simulink model "quad_ASMC"  (R2023a)
settings: Solver=ode4  StartTime=0.0  StopTime=tf  FixedStep=0.01  RelTol=1e-3
model workspace (MAT data in the model file):
  tf = Simulink.Parameter
  tf.Value = 60
  tf.DataType = 'auto'
  tf.Complexity = 'real'
  tf.Dimensions = [1 1]
  tray2 = [0  2  2  -2  -2  0; 0  0  -2  -2  2  0; 0  5  2.5  5  2.5  0; 0  0  0  0  0  0; 0  0  0  0  0  0; 0  0  0  0  0  0]
libraries: robotcorelib x1
settings Model: Creator=adan  LastModifiedBy=Adan Daniel
settings OptimizationCC: ReuseModelBlockBuffer=off

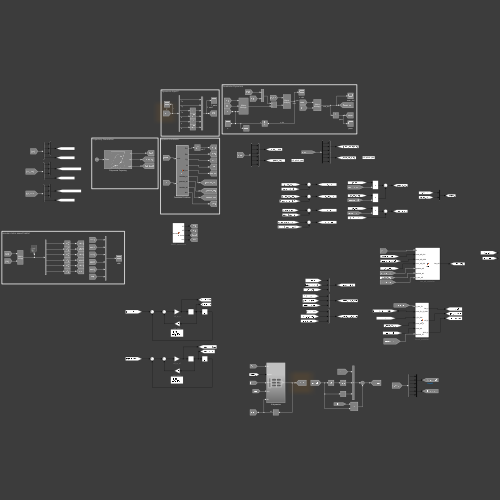
[thumbnail: Simulink's stored preview of the top-level diagram]
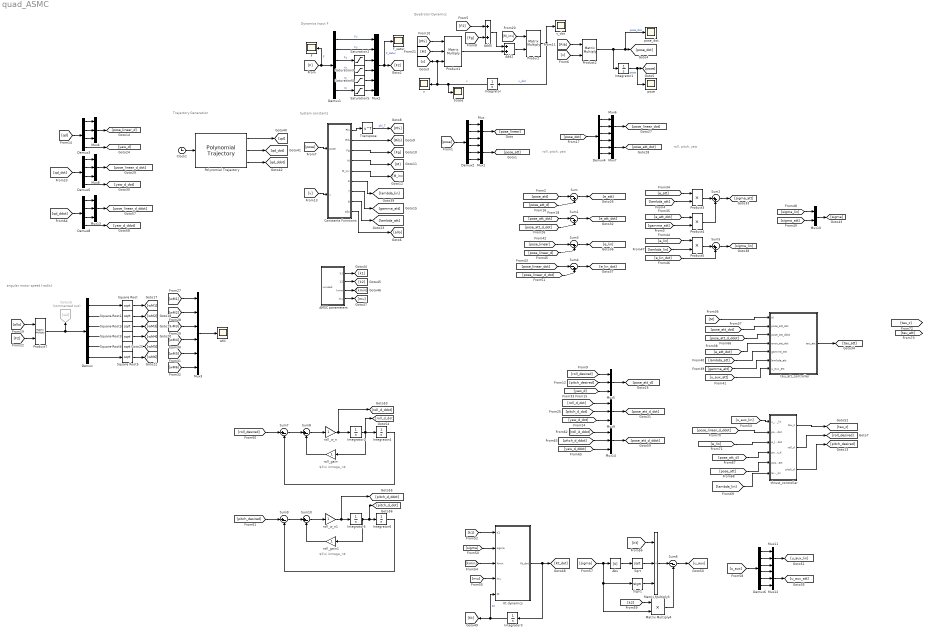
== system quad_ASMC ==
  note: $2\xi \omega_n$
  note: roll, pitch, yaw
  note: angular motor speed [rad/s]
  note: System constants
  note: Quadrotor Dynamics
  note: Dynamics Input F
  note: Trajectory Generation
  note: roll, pitch, yaw
  note: $2\xi \omega_n$
  AMSC parameters : MATLAB Function  TreatAsAtomicUnit=on
  Abs : Abs  SaturateOnIntegerOverflow=off
  Add2 : Sum
  Add5 : Sum
  Clock1 : Clock
  Constants Functions : MATLAB Function  TreatAsAtomicUnit=on
  Demux{,1..2,4,6} (5 alike) : Demux  Outputs=6
  Demux3 : Demux
  Demux5 : Demux
  Demux8 : Demux
  F : Scope
  F_satur : Scope
  Goto16 : Goto  Commented=on  GotoTag=w2
  Integrator : Integrator  InitialCondition=[0; 0; 0; 0; 0; 0]
  Integrator1 : Integrator  InitialCondition=[0; 0; 0; 0; 0; 0]
  Integrator{2,4..6} (4 alike) : Integrator
  Integrator3 : Integrator  InitialCondition=[0; 0; 0; 0; 0; 0]
  Kt dynamics : Subsystem
  Matrix Multiply3 : Product  Inputs=3
  Matrix Multiply4 : Product
  Mux{,1,4..9,11..14} (12 alike) : Mux  Inputs=3
  Mux10 : Mux  Inputs=2
  Mux2 : Mux  Inputs=6
  Mux3 : Mux  Inputs=6
  Polynomial Trajectory : robotcorelib/Polynomial Trajectory  WaypointSource=Internal  Waypoints=tray2  TimePoints=[ 0, 12, 24, 35, 48, tf ]  TimeInterval=[ 1, 4 ]  Method=Cubic Polynomial  ParameterSource=Internal  VelocityBoundaryCondition=zeros( 6, 6 )  AccelerationBoundaryCondition=zeros( 2, 5 )  SimulateUsing=Interpreted execution
  Product : Product  Multiplication=Matrix(*)
  Product1 : Product  Inputs=3  Multiplication=Matrix(*)
  Product2 : Product  Multiplication=Matrix(*)
  Product3 : Product
  Product4 : Product
  Product5 : Product
  Product7 : Product  Multiplication=Matrix(*)
  Saturation2 : Saturate  UpperLimit=5.8*6  LowerLimit=0
  Saturation3 : Saturate
  Saturation4 : Saturate
  Saturation5 : Saturate
  Scope : Scope
  Sign1 : Signum
  Sqrt : Sqrt
  Square Root{,1..5} (6 alike) : Sqrt
  Sum{,1,3..4} (4 alike) : Sum  Inputs=|-+
  Sum{7..10} (4 alike) : Sum  Inputs=|+-
  Sum2 : Sum  Inputs=|++
  Sum5 : Sum  Inputs=|++
  Sum6 : Sum  Inputs=|--
  Transpose : Math  Operator=transpose
  pose : Scope
  pose_dot : Scope
  roll_gain : Gain
  roll_gain1 : Gain
  roll_w_n : Gain
  roll_w_n1 : Gain
  tau_att_controller : MATLAB Function  TreatAsAtomicUnit=on
  thrust_controller : MATLAB Function  TreatAsAtomicUnit=on
  v : Scope
  v_dot : Scope
  wMi : Scope
  wires:
  Saturation4/1 -> Mux2/5
  Saturation3/1 -> Mux2/4
  Demux1/6 -> Saturation5/1  "tz"
  Demux1/3 -> Saturation2/1  "Fz"
  [F] -> F/1, Demux1/1  "F"
  Saturation5/1 -> Mux2/6
  Demux1/2 -> Mux2/2  "Fy"
  Demux1/1 -> Mux2/1  "Fx"
  Demux1/5 -> Saturation4/1  "ty"
  Demux1/4 -> Saturation3/1  "tx"
  Saturation2/1 -> Mux2/3
  Mux2/1 -> F_satur/1, [F2]  "F_satur"
  [M] -> Product1/2
  [v] -> Product2/2
  [M_inv] -> Product/1
  Add2/1 -> Product/2
  Product/1 -> v_dot/1, Integrator/1  "v_dot"
  [Rib] -> Product2/1
  Product2/1 -> Integrator1/1, pose_dot/1, [pose_dot]  "pose_dot"
  [Phi] -> Product1/1
  Product1/1 -> Add2/2
  Integrator1/1 -> pose/1, [pose]  "pose"
  Integrator/1 -> Scope/1, v/1, [v], Product1/3  "v"
  [Fg] -> Add5/2
  Add5/1 -> Add2/1
  [F2] -> Add5/1
  Constants Functions/1(Phi) -> Transpose/1
  Constants Functions/3(Fg) -> [Fg]
  Constants Functions/2(Rib) -> [Rib]
  Transpose/1 -> [Phi]  "phi_T"
  Constants Functions/5(M_inv) -> [M_inv]
  Constants Functions/4(M) -> [M]
  Constants Functions/9(allo) -> [allo]
  [v] -> Constants Functions/2(v)
  [pose] -> Constants Functions/1(pose)
  [wM3] -> Mux3/3
  [allo] -> Product7/1
  [wM6] -> Mux3/6
  [wM2] -> Mux3/2
  Demux/2 -> Square Root1/1
  Product7/1 -> Demux/1, Goto16/1
  Demux/6 -> Square Root5/1
  Demux/5 -> Square Root4/1
  [wM4] -> Mux3/4
  Mux3/1 -> wMi/1
  Square Root2/1 -> [wM3]
  Demux/4 -> Square Root3/1
  Demux/1 -> Square Root/1
  [wM1] -> Mux3/1
  [F2] -> Product7/2
  Square Root1/1 -> [wM2]
  [wM5] -> Mux3/5
  Square Root4/1 -> [wM5]
  Demux/3 -> Square Root2/1
  Square Root5/1 -> [wM6]
  Square Root3/1 -> [wM4]
  Square Root/1 -> [wM1]
  Polynomial Trajectory/1 -> [qd]
  Clock1/1 -> Polynomial Trajectory/1
  Polynomial Trajectory/2 -> [qd_dot]
  Polynomial Trajectory/3 -> [qd_ddot]
  Constants Functions/7(gamma_att) -> [gamma_att]
  Constants Functions/8(lambda_att) -> [lambda_att]
  [pose] -> Demux2/1
  Demux2/3 -> Mux/3
  Demux2/2 -> Mux/2
  Demux2/1 -> Mux/1
  Demux2/4 -> Mux1/1
  Demux2/5 -> Mux1/2
  Demux2/6 -> Mux1/3
  Mux/1 -> [pose_linear]
  Mux1/1 -> [pose_att]
  [qd] -> Demux3/1
  Demux3/3 -> Mux4/3
  Demux3/2 -> Mux4/2
  Demux3/1 -> Mux4/1
  Mux4/1 -> [pose_linear_d]
  Demux3/4 -> [yaw_d]
  [yaw_d] -> Mux5/3
  [pitch_desired] -> Mux5/2
  [roll_desired] -> Mux5/1
  Mux5/1 -> [pose_att_d]
  [pose_att] -> Sum/1
  [pose_att_d] -> Sum/2
  Sum/1 -> [e_att]
  Mux7/1 -> [pose_att_dot]
  Demux4/6 -> Mux7/3
  [pose_dot] -> Demux4/1
  Demux4/1 -> Mux6/1
  Demux4/2 -> Mux6/2
  Demux4/5 -> Mux7/2
  Demux4/4 -> Mux7/1
  Mux6/1 -> [pose_linear_dot]
  Demux4/3 -> Mux6/3
  Demux5/2 -> Mux8/2
  Mux8/1 -> [pose_linear_d_dot]
  Demux5/4 -> [yaw_d_dot]
  [qd_dot] -> Demux5/1
  Demux5/3 -> Mux8/3
  Demux5/1 -> Mux8/1
  [pitch_d_dot] -> Mux9/2
  [yaw_d_dot] -> Mux9/3
  Mux9/1 -> [pose_att_d_dot]
  [roll_d_dot] -> Mux9/1
  [pose_att_d_dot] -> Sum1/2
  [pose_att_dot] -> Sum1/1
  Sum1/1 -> [e_att_dot]
  [e_att] -> Product3/1
  [lambda_att] -> Product3/2
  [gamma_att] -> Product4/2
  [e_att_dot] -> Product4/1
  Product3/1 -> Sum2/1
  Product4/1 -> Sum2/2
  Sum2/1 -> [sigma_att]
  [M] -> tau_att_controller/1(M)
  [pose_att_dot] -> tau_att_controller/2(pose_att_dot)
  [e_att_dot] -> tau_att_controller/4(error_att_dot)
  [lambda_att] -> tau_att_controller/5(gamma_att)
  [gamma_att] -> tau_att_controller/6(lambda_att)
  [u_aux_att] -> tau_att_controller/7(u_aux_att)
  tau_att_controller/1(tau_att) -> [tau_att]
  Sum4/1 -> [e_lin_dot]
  [e_lin_dot] -> Sum5/2
  [pose_linear_d] -> Sum3/2
  [lambda_lin] -> Product5/2
  [e_lin] -> Product5/1
  [pose_linear_dot] -> Sum4/1
  [pose_linear_d_dot] -> Sum4/2
  Product5/1 -> Sum5/1
  [pose_linear] -> Sum3/1
  Sum5/1 -> [sigma_lin]
  Sum3/1 -> [e_lin]
  Constants Functions/6(lambda_lin) -> [lambda_lin]
  [sigma_lin] -> Mux10/1
  [sigma_att] -> Mux10/2
  Mux10/1 -> [sigma]
  AMSC parameters/1(k1) -> [k1]
  AMSC parameters/2(k2) -> [k2]
  AMSC parameters/3(kmin) -> [kmin]
  AMSC parameters/4(mu) -> [mu]
  [sigma] -> Kt dynamics/2(sigma)
  [k1] -> Kt dynamics/1(K1)
  [mu] -> Kt dynamics/4(mu)
  [kmin] -> Kt dynamics/3(Kmin)
  Kt dynamics/1(Kt_dot) -> Integrator3/1, [Kt_dot]
  Integrator3/1 -> [Kt], Kt dynamics/5(Kt)  "Kt"
  Sqrt/1 -> Matrix Multiply3/2
  Sum6/1 -> [u_aux]
  Matrix Multiply3/1 -> Sum6/1
  Matrix Multiply4/1 -> Sum6/2
  Abs/1 -> Sqrt/1
  Sign1/1 -> Matrix Multiply3/3
  [sigma] -> Matrix Multiply4/2, Sign1/1, Abs/1
  [k2] -> Matrix Multiply4/1
  [Kt] -> Matrix Multiply3/1
  Mux12/1 -> [u_aux_att]
  Demux6/6 -> Mux12/3
  [u_aux] -> Demux6/1
  Demux6/1 -> Mux11/1
  Demux6/2 -> Mux11/2
  Demux6/5 -> Mux12/2
  Demux6/4 -> Mux12/1
  Mux11/1 -> [u_aux_lin]
  Demux6/3 -> Mux11/3
  [roll_desired] -> Sum7/1
  Sum7/1 -> Sum8/1
  Sum8/1 -> roll_w_n/1
  roll_w_n/1 -> [roll_d_ddot], Integrator2/1
  Integrator2/1 -> Integrator4/1, roll_gain/1, [roll_d_dot]
  roll_gain/1 -> Sum8/2
  Integrator4/1 -> Sum7/2
  roll_gain1/1 -> Sum10/2
  [pitch_desired] -> Sum9/1
  Integrator5/1 -> roll_gain1/1, [pitch_d_dot], Integrator6/1
  Sum9/1 -> Sum10/1
  Integrator6/1 -> Sum9/2
  roll_w_n1/1 -> [pitch_d_ddot], Integrator5/1
  Sum10/1 -> roll_w_n1/1
  Mux13/1 -> [pose_linear_d_ddot]
  Demux8/4 -> [yaw_d_ddot]
  Demux8/1 -> Mux13/1
  [qd_ddot] -> Demux8/1
  Demux8/3 -> Mux13/3
  Demux8/2 -> Mux13/2
  [roll_d_ddot] -> Mux14/1
  [yaw_d_ddot] -> Mux14/3
  Mux14/1 -> [pose_att_d_ddot]
  [pitch_d_ddot] -> Mux14/2
  [pose_att_d_ddot] -> tau_att_controller/3(pose_att_ddot)
  [u_aux_lin] -> thrust_controller/1(u_aux_lin)
  [pose_att_d] -> thrust_controller/4(pose_att_d)
  thrust_controller/3(pitch_d) -> [pitch_desired]
  thrust_controller/2(roll_d) -> [roll_desired]
  thrust_controller/1(tau_z) -> [tau_z]
  [pose_att] -> thrust_controller/5(pose_att)
  [lambda_lin] -> thrust_controller/6(lambda_lin)
  [pose_linear_d_ddot] -> thrust_controller/2(pose_lin_d_ddot)
  [e_lin] -> thrust_controller/3(e_lin_dot)

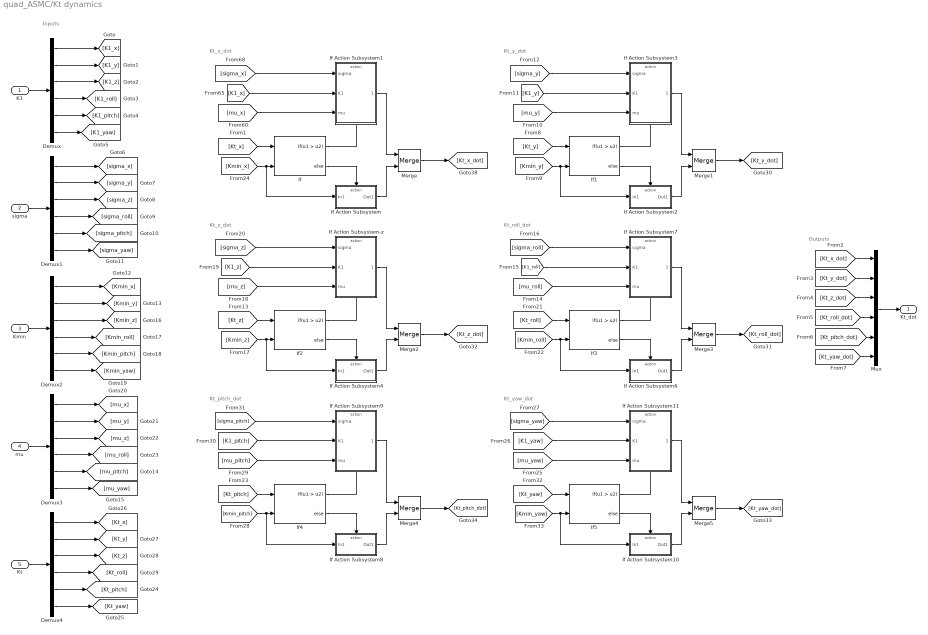
== system quad_ASMC/Kt dynamics ==
  note: Outputs
  note: Inputs
  note: Kt_x_dot
  note: Kt_y_dot
  note: Kt_z_dot
  note: Kt_roll_dot
  note: Kt_pitch_dot
  note: Kt_yaw_dot
  K1 : Inport
  sigma : Inport  Port=2
  Kmin : Inport  Port=3
  mu : Inport  Port=4
  Kt : Inport  Port=5
  Demux{,1..4} (5 alike) : Demux  Outputs=6
  If{,1..5} (6 alike) : If  NumInputs=2  IfExpression=u1 > u2
  If Action Subsystem : Subsystem  TreatAsAtomicUnit=on
  If Action Subsystem-z : Subsystem  TreatAsAtomicUnit=on
  If Action Subsystem1 : Subsystem  TreatAsAtomicUnit=on
  If Action Subsystem10 : Subsystem  TreatAsAtomicUnit=on
  If Action Subsystem11 : Subsystem  TreatAsAtomicUnit=on
  If Action Subsystem2 : Subsystem  TreatAsAtomicUnit=on
  If Action Subsystem3 : Subsystem  TreatAsAtomicUnit=on
  If Action Subsystem4 : Subsystem  TreatAsAtomicUnit=on
  If Action Subsystem6 : Subsystem  TreatAsAtomicUnit=on
  If Action Subsystem7 : Subsystem  TreatAsAtomicUnit=on
  If Action Subsystem8 : Subsystem  TreatAsAtomicUnit=on
  If Action Subsystem9 : Subsystem  TreatAsAtomicUnit=on
  Merge{,1..5} (6 alike) : Merge
  Mux : Mux  Inputs=6
  Kt_dot : Outport
  wires:
  [Kt_x] -> If/1
  [sigma_x] -> If Action Subsystem1/1(sigma)
  If/1 -> If Action Subsystem1/Action
  [K1_x] -> If Action Subsystem1/2(K1)
  If Action Subsystem1/1(Kt_x_dot) -> Merge/1
  If Action Subsystem/1(Out1) -> Merge/2
  If/2 -> If Action Subsystem/Action
  Merge/1 -> [Kt_x_dot]
  [Kmin_x] -> If Action Subsystem/1(In1), If/2
  [mu_x] -> If Action Subsystem1/3(mu)
  Merge1/1 -> [Kt_y_dot]
  If1/2 -> If Action Subsystem2/Action
  If Action Subsystem2/1(Out1) -> Merge1/2
  If Action Subsystem3/1(Kt_x_dot) -> Merge1/1
  [Kt_y] -> If1/1
  [K1_y] -> If Action Subsystem3/2(K1)
  [mu_y] -> If Action Subsystem3/3(mu)
  [Kmin_y] -> If Action Subsystem2/1(In1), If1/2
  [sigma_y] -> If Action Subsystem3/1(sigma)
  Merge2/1 -> [Kt_z_dot]
  If Action Subsystem-z/1(Kt_z_dot) -> Merge2/1
  [sigma_z] -> If Action Subsystem-z/1(sigma)
  [Kt_z] -> If2/1
  [mu_z] -> If Action Subsystem-z/3(mu)
  [Kmin_z] -> If Action Subsystem4/1(In1), If2/2
  If3/2 -> If Action Subsystem6/Action
  If Action Subsystem7/1(Kt_x_dot) -> Merge3/1
  Merge3/1 -> [Kt_roll_dot]
  If3/1 -> If Action Subsystem7/Action
  [Kmin_roll] -> If Action Subsystem6/1(In1), If3/2
  If2/2 -> If Action Subsystem4/Action
  [sigma_roll] -> If Action Subsystem7/1(sigma)
  If2/1 -> If Action Subsystem-z/Action
  [K1_roll] -> If Action Subsystem7/2(K1)
  If Action Subsystem6/1(Out1) -> Merge3/2
  [mu_roll] -> If Action Subsystem7/3(mu)
  If Action Subsystem4/1(Out1) -> Merge2/2
  [Kt_roll] -> If3/1
  [K1_z] -> If Action Subsystem-z/2(K1)
  Merge4/1 -> [Kt_pitch_dot]
  If Action Subsystem9/1(Kt_x_dot) -> Merge4/1
  [sigma_pitch] -> If Action Subsystem9/1(sigma)
  [Kt_pitch] -> If4/1
  [mu_pitch] -> If Action Subsystem9/3(mu)
  [Kmin_pitch] -> If Action Subsystem8/1(In1), If4/2
  If5/2 -> If Action Subsystem10/Action
  If Action Subsystem11/1(Kt_x_dot) -> Merge5/1
  Merge5/1 -> [Kt_yaw_dot]
  If5/1 -> If Action Subsystem11/Action
  [Kmin_yaw] -> If Action Subsystem10/1(In1), If5/2
  If4/2 -> If Action Subsystem8/Action
  [sigma_yaw] -> If Action Subsystem11/1(sigma)
  If4/1 -> If Action Subsystem9/Action
  [K1_yaw] -> If Action Subsystem11/2(K1)
  If Action Subsystem10/1(Out1) -> Merge5/2
  [mu_yaw] -> If Action Subsystem11/3(mu)
  If Action Subsystem8/1(Out1) -> Merge4/2
  [Kt_yaw] -> If5/1
  [K1_pitch] -> If Action Subsystem9/2(K1)
  If1/1 -> If Action Subsystem3/Action
  Demux4/6 -> [Kt_yaw]
  Demux4/1 -> [Kt_x]
  Demux1/5 -> [sigma_pitch]
  Demux1/3 -> [sigma_z]
  Demux1/1 -> [sigma_x]
  Demux1/2 -> [sigma_y]
  Kt/1 -> Demux4/1
  Demux4/4 -> [Kt_roll]
  sigma/1 -> Demux1/1
  Demux3/4 -> [mu_roll]
  Demux2/4 -> [Kmin_roll]
  Demux3/1 -> [mu_x]
  Demux2/3 -> [Kmin_z]
  Demux3/3 -> [mu_z]
  mu/1 -> Demux3/1
  Demux3/6 -> [mu_yaw]
  Demux3/5 -> [mu_pitch]
  Demux2/5 -> [Kmin_pitch]
  Demux3/2 -> [mu_y]
  Demux2/6 -> [Kmin_yaw]
  Demux2/1 -> [Kmin_x]
  Demux2/2 -> [Kmin_y]
  Demux/4 -> [K1_roll]
  Demux1/4 -> [sigma_roll]
  Demux4/5 -> [Kt_pitch]
  Demux4/2 -> [Kt_y]
  Demux4/3 -> [Kt_z]
  Demux/1 -> [K1_x]
  K1/1 -> Demux/1
  Demux/6 -> [K1_yaw]
  Demux/5 -> [K1_pitch]
  Demux1/6 -> [sigma_yaw]
  Demux/2 -> [K1_y]
  Kmin/1 -> Demux2/1
  Demux/3 -> [K1_z]
  Mux/1 -> Kt_dot/1
  [Kt_z_dot] -> Mux/3
  [Kt_yaw_dot] -> Mux/6
  [Kt_pitch_dot] -> Mux/5
  [Kt_x_dot] -> Mux/1
  [Kt_y_dot] -> Mux/2
  [Kt_roll_dot] -> Mux/4

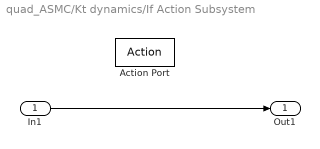
== system quad_ASMC/Kt dynamics/If Action Subsystem ==
  In1 : Inport
  Action Port : ActionPort
  Out1 : Outport
  wires:
  In1/1 -> Out1/1

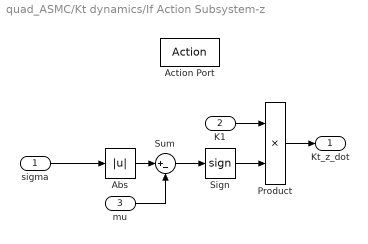
== system quad_ASMC/Kt dynamics/If Action Subsystem-z ==
  sigma : Inport
  K1 : Inport  Port=2
  mu : Inport  Port=3
  Action Port : ActionPort
  Abs : Abs  SaturateOnIntegerOverflow=off
  Product : Product
  Sign : Signum
  Sum : Sum  Inputs=|+-
  Kt_z_dot : Outport
  wires:
  sigma/1 -> Abs/1
  Abs/1 -> Sum/1
  mu/1 -> Sum/2
  Sum/1 -> Sign/1
  Product/1 -> Kt_z_dot/1
  Sign/1 -> Product/2
  K1/1 -> Product/1

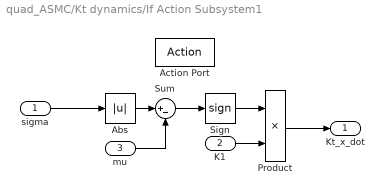
== system quad_ASMC/Kt dynamics/If Action Subsystem1 ==
  sigma : Inport
  K1 : Inport  Port=2
  mu : Inport  Port=3
  Action Port : ActionPort
  Abs : Abs  SaturateOnIntegerOverflow=off
  Product : Product
  Sign : Signum
  Sum : Sum  Inputs=|+-
  Kt_x_dot : Outport
  wires:
  sigma/1 -> Abs/1
  Abs/1 -> Sum/1
  mu/1 -> Sum/2
  Sum/1 -> Sign/1
  Sign/1 -> Product/1
  K1/1 -> Product/2
  Product/1 -> Kt_x_dot/1

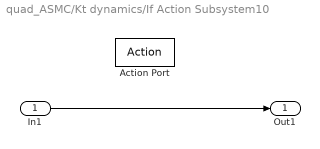
== system quad_ASMC/Kt dynamics/If Action Subsystem10 ==
  In1 : Inport
  Action Port : ActionPort
  Out1 : Outport
  wires:
  In1/1 -> Out1/1

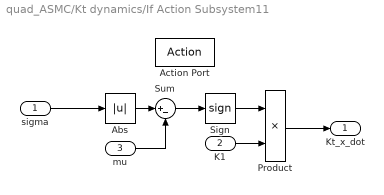
== system quad_ASMC/Kt dynamics/If Action Subsystem11 ==
  sigma : Inport
  K1 : Inport  Port=2
  mu : Inport  Port=3
  Action Port : ActionPort
  Abs : Abs  SaturateOnIntegerOverflow=off
  Product : Product
  Sign : Signum
  Sum : Sum  Inputs=|+-
  Kt_x_dot : Outport
  wires:
  sigma/1 -> Abs/1
  Abs/1 -> Sum/1
  mu/1 -> Sum/2
  Sum/1 -> Sign/1
  Sign/1 -> Product/1
  K1/1 -> Product/2
  Product/1 -> Kt_x_dot/1

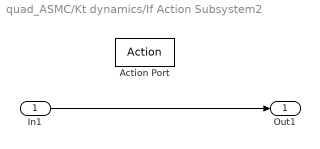
== system quad_ASMC/Kt dynamics/If Action Subsystem2 ==
  In1 : Inport
  Action Port : ActionPort
  Out1 : Outport
  wires:
  In1/1 -> Out1/1

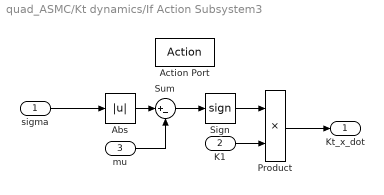
== system quad_ASMC/Kt dynamics/If Action Subsystem3 ==
  sigma : Inport
  K1 : Inport  Port=2
  mu : Inport  Port=3
  Action Port : ActionPort
  Abs : Abs  SaturateOnIntegerOverflow=off
  Product : Product
  Sign : Signum
  Sum : Sum  Inputs=|+-
  Kt_x_dot : Outport
  wires:
  sigma/1 -> Abs/1
  Abs/1 -> Sum/1
  mu/1 -> Sum/2
  Sum/1 -> Sign/1
  Sign/1 -> Product/1
  K1/1 -> Product/2
  Product/1 -> Kt_x_dot/1

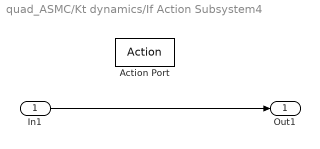
== system quad_ASMC/Kt dynamics/If Action Subsystem4 ==
  In1 : Inport
  Action Port : ActionPort
  Out1 : Outport
  wires:
  In1/1 -> Out1/1

== system quad_ASMC/Kt dynamics/If Action Subsystem6 ==
  In1 : Inport
  Action Port : ActionPort
  Out1 : Outport
  wires:
  In1/1 -> Out1/1

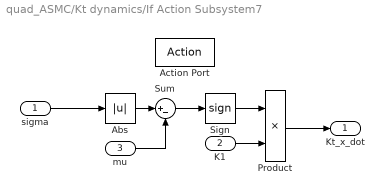
== system quad_ASMC/Kt dynamics/If Action Subsystem7 ==
  sigma : Inport
  K1 : Inport  Port=2
  mu : Inport  Port=3
  Action Port : ActionPort
  Abs : Abs  SaturateOnIntegerOverflow=off
  Product : Product
  Sign : Signum
  Sum : Sum  Inputs=|+-
  Kt_x_dot : Outport
  wires:
  sigma/1 -> Abs/1
  Abs/1 -> Sum/1
  mu/1 -> Sum/2
  Sum/1 -> Sign/1
  Sign/1 -> Product/1
  K1/1 -> Product/2
  Product/1 -> Kt_x_dot/1

== system quad_ASMC/Kt dynamics/If Action Subsystem8 ==
  In1 : Inport
  Action Port : ActionPort
  Out1 : Outport
  wires:
  In1/1 -> Out1/1

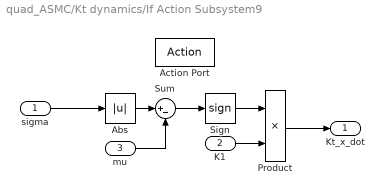
== system quad_ASMC/Kt dynamics/If Action Subsystem9 ==
  sigma : Inport
  K1 : Inport  Port=2
  mu : Inport  Port=3
  Action Port : ActionPort
  Abs : Abs  SaturateOnIntegerOverflow=off
  Product : Product
  Sign : Signum
  Sum : Sum  Inputs=|+-
  Kt_x_dot : Outport
  wires:
  sigma/1 -> Abs/1
  Abs/1 -> Sum/1
  mu/1 -> Sum/2
  Sum/1 -> Sign/1
  Sign/1 -> Product/1
  K1/1 -> Product/2
  Product/1 -> Kt_x_dot/1

== matlab function quad_ASMC/AMSC parameters ==
  data: unused input; k1 output; k2 output; kmin output; mu output
function [k1, k2, kmin, mu]= fcn(~)

k1 = [1;
      1;
      1;
      1;
      1;
      1];

k2 = [1;
      1;
      1;
      1;
      1;
      1];

kmin = [1;
      1;
      1;
      1;
      1;
      1];

mu = [0.01;
      0.01;
      0.01;
      0.01;
      0.01;
      0.01];

== matlab function quad_ASMC/tau_att_controller ==
  data: M input; pose_att_dot input; pose_att_ddot input; tau_att output; error_att_dot input; gamma_att input; lambda_att input; u_aux_att input
function tau_att = fcn(M, pose_att_dot, pose_att_ddot, error_att_dot, gamma_att, lambda_att, u_aux_att)

l = 0.25;

% Inertial values

Jxx = M(4,4);
Jyy = M(5,5);
Jzz = M(6,6);

%pose dot values

roll_dot = pose_att_dot(1);
pitch_dot = pose_att_dot(2); 
yaw_dot = pose_att_dot(3);

% pose desired ddot 

roll_d_ddot = pose_att_ddot(1);
pitch_d_ddot = pose_att_ddot(2);
yaw_d_ddot = pose_att_ddot(3);

%% Constant definitions

a1 = ((Jyy - Jzz)/Jxx)*(pitch_dot * yaw_dot);
a2 = ((Jzz - Jxx)/Jyy)*(roll_dot * yaw_dot);
a3 = ((Jxx - Jyy)/Jzz)*(roll_dot * pitch_dot);

b1 = l/Jxx;
b2 = l/Jyy;
b3 = 1/Jzz;

%% attitude controller

tau_roll = (1/(gamma_att(1) * b1)) * ((gamma_att(1) * roll_d_ddot) - lambda_att(1) * error_att_dot(1) - gamma_att(1) * a1 + u_aux_att(1));
tau_pitch = (1/(gamma_att(2) * b2)) * ((gamma_att(2) * pitch_d_ddot) - lambda_att(2) * error_att_dot(2) - gamma_att(2) * a2 + u_aux_att(2));
tau_yaw = (1/(gamma_att(3) * b3)) * ((gamma_att(3) * yaw_d_ddot) - lambda_att(3) * error_att_dot(3) - gamma_att(3) * a3 + u_aux_att(3));


%% tau

tau_att = [tau_roll; tau_pitch; tau_yaw];

== matlab function quad_ASMC/Constants Functions ==
  data: Phi output; Rib output; Fg output; pose input; M output; M_inv output; lambda_lin output; gamma_att output; lambda_att output; v input; allo output
function [Phi, Rib, Fg, M, M_inv, lambda_lin, gamma_att, lambda_att, allo]   = fcn(pose, v)

%% System constants
m = 1.525; %5 mass 2.2 kg
l = 0.25; % m
g = 9.81; % gravity
Jxx =  0.0411; % kg m²
Jyy = 0.0478; % kg m²
Jzz = 0.0599; % kg m²
kT = 3.4e-5;
kQ = 3.4e-6;
%% Phi vector 6d

uu = v(1);
vv = v(2);
ww = v(3);
pp = v(4);
qq = v(5);
rr = v(6);


Phi = [0, -rr, qq, 0, -ww, vv;
        rr, 0, -pp , ww, 0, -uu;
        -qq, pp, 0,  -vv, uu, 0;
        0, 0, 0, 0, -rr, qq; 
        0, 0, 0, rr, 0, -pp;
        0, 0, 0, -qq, pp, 0];
%% Fg and Rib calculation

roll = pose(4);
pitch = pose(5);
yaw = pose(6);


Rib = [cos(yaw)*cos(pitch), -cos(roll)*sin(yaw) + cos(yaw)*sin(roll)*sin(pitch), sin(roll)*sin(yaw) + cos(roll)*cos(yaw)*sin(pitch), 0, 0, 0;
       cos(pitch)*sin(yaw), cos(roll)*cos(yaw) + sin(yaw)*sin(pitch)*sin(roll), -cos(yaw)*sin(roll) + sin(yaw)*sin(pitch)*cos(roll), 0, 0, 0;
       -sin(pitch), cos(pitch)*sin(roll), cos(pitch)*cos(roll), 0, 0, 0;
       0, 0, 0, 1, sin(roll)*tan(pitch), cos(roll)*tan(pitch);
       0, 0, 0, 0, cos(roll), -sin(roll);
       0, 0, 0, 0, sin(roll)/cos(pitch), cos(roll)/cos(pitch)];

Fg = [m*g*sin(pitch);
      -m*g*cos(pitch)*sin(roll);
      -m*g*cos(pitch)*cos(roll);
      0;
      0;
      0];

%% M matrix

M = [m, 0, 0, 0, 0, 0;
    0, m, 0, 0, 0, 0;
    0, 0, m, 0, 0, 0;
    0, 0, 0, Jxx, 0, 0;
    0, 0, 0, 0, Jyy, 0;
    0, 0, 0, 0, 0, Jzz];

M_inv = inv(M);

%% Allocation matrix

allo = [0, 0, 0, 0, 0, 0;
        0, 0, 0, 0, 0, 0;
        kT, kT, kT, kT, kT, kT;
        -kT*l, kT*l, kT*l/2, -kT*l/2, -kT*l/2, kT*l/2;
        0, 0, -sqrt(3)*kT*l/2, sqrt(3)*kT*l/2, -sqrt(3)*kT*l/2, sqrt(3)*kT*l/2;
        kQ, -kQ, kQ, -kQ, -kQ, kQ,];

allo = pinv(allo);

lambda_lin = [2; 2; 2];

gamma_att = [1; 1; 1];

lambda_att = [2; 2; 2];

== matlab function quad_ASMC/thrust_controller ==
  data: u_aux_lin input; pose_lin_d_ddot input; e_lin_dot input; tau_z output; pose_att_d input; roll_d output; pitch_d output; pose_att input; lambda_lin input
function [tau_z, roll_d, pitch_d] = fcn(u_aux_lin, pose_lin_d_ddot, e_lin_dot, pose_att_d, pose_att, lambda_lin)

% variables

m = 1.525;
g = 9.81;
lambda_z = lambda_lin(3);
z_d_ddot = pose_lin_d_ddot(3);

roll_d = pose_att_d(1);
%pitch_d = pose_att_d(2);
yaw_d = pose_att_d(3);

roll = pose_att(1);
pitch = pose_att(2);

%% thrust calculation

tau_z = (m/cos(pitch)*cos(roll)) * (u_aux_lin(3) - g) + z_d_ddot - lambda_z * (e_lin_dot(3));

%% roll & pitch desired

roll_des_calculation = (m/tau_z) * (sin(roll_d) * u_aux_lin(1) - cos(yaw_d) * u_aux_lin(2));

if roll_des_calculation > 1
    roll_des_calculation = 1;
elseif roll_des_calculation < -1
    roll_des_calculation = -1;
end
roll_d = asin(roll_des_calculation);

pitch_des_calculation = (m*u_aux_lin(1)/tau_z - sin(yaw_d) * sin(roll_d))/(cos(yaw_d) * cos(roll_d));

if (pitch_des_calculation > 1)
    pitch_des_calculation = 1;
elseif (pitch_des_calculation < -1)
    pitch_des_calculation = -1;
end

pitch_d = asin(pitch_des_calculation);
